simulink model "fan_controller"  (R2020a)
settings: Solver=FixedStepDiscrete  StartTime=0.0  StopTime=10.0  FixedStep=1  RelTol=1e-3
model workspace (MAT data in the model file):
  initial_h = Simulink.Parameter
  initial_h.Value = 50
  initial_h.Description = 'Initial humidity value to preload downsamplers and differentiators/integrators'
  initial_h.DataType = 'auto'
  initial_h.DocUnits = '%'
  initial_h.Dimensions = [1 1]
  initial_t = Simulink.Parameter
  initial_t.Value = 25
  initial_t.Description = 'Initial temperature value to preload downsamplers and differentiators/integrators'
  initial_t.DataType = 'auto'
  initial_t.DocUnits = '°C'
  initial_t.Dimensions = [1 1]
libraries: dspstat3 x4, simulink x2
settings Model: DataDictionary=fan_controller_setup.sldd  OrderedModelArguments=off  Creator=Kalev  LastModifiedBy=Kalev
settings OptimizationCC: EnhancedBackFolding=on  PassReuseOutputArgsAs=Individual arguments  ZeroExternalMemoryAtStartup=off  ZeroInternalMemoryAtStartup=off  OptimizeBlockOrder=speed  DifferentSizesBufferReuse=on  OptimizationCustomize=off  EfficientTunableParamExpr=on
settings DebuggingCC: ParameterTunabilityLossMsg=error
settings HardwareCC: ProdBitPerPointer=32  ProdBitPerSizeT=32  ProdBitPerPtrDiffT=32  ProdLargestAtomicInteger=Integer  ProdLargestAtomicFloat=Double  ProdWordSize=32  ProdHWDeviceType=Custom Processor->Custom Processor
settings SFSimCC: MATLABDynamicMemAlloc=off
settings RTWCC: SystemTargetFile=ert.tlc  GenCodeOnly=on  TemplateMakefile=ert_default_tmf  GenerateReport=on  BuildConfiguration=Debug  LaunchReport=on  TargetLang=C++
settings CodeAppCC: ForceParamTrailComments=on  IgnoreCustomStorageClasses=off  OperatorAnnotations=on  SimulinkDataObjDesc=on  SFDataObjDesc=on  InsertBlockDesc=on
settings ERTTargetCC: TargetLangStandard=C++03 (ISO)  GenerateSampleERTMain=on  MultiInstanceERTCode=on  CodeInterfacePackaging=C++ class  RootIOFormat=Structure reference  ERTCustomFileTemplate=example_file_process.tlc

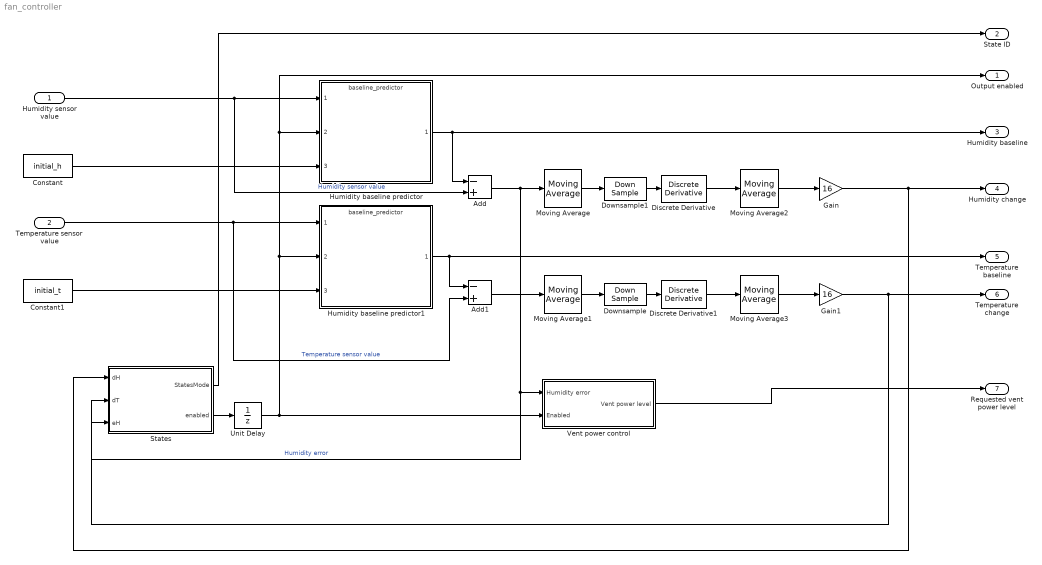
== system fan_controller ==
  Humidity sensor value : Inport
  Temperature sensor value : Inport  Port=2
  Add : Sum  Inputs=-+
  Add1 : Sum  Inputs=-+
  Constant : Constant  Value=initial_h
  Constant1 : Constant  Value=initial_t
  Discrete Derivative : simulink/Discrete/Discrete Derivative  gainval=1.0  ICPrevScaledInput=initial_h  OutMin=[]  OutMax=[]  OutDataType=fixdt(1, 16)  OutScaling=2^-10  DoSatur=off
  Discrete Derivative1 : simulink/Discrete/Discrete Derivative  gainval=1.0  ICPrevScaledInput=initial_t  OutMin=[]  OutMax=[]  OutDataType=fixdt(1, 16)  OutScaling=2^-10  DoSatur=off
  Downsample : DownSample  N=16  phase=15  ic=initial_t
  Downsample1 : DownSample  N=16  phase=15  ic=initial_h
  Gain : Gain  Gain=16
  Gain1 : Gain  Gain=16
  Humidity baseline predictor : ModelReference  ModelNameDialog=baseline_predictor.slx  SimulationMode=Normal  ModelReferenceVersion=1.4
  Humidity baseline predictor1 : ModelReference  ModelNameDialog=baseline_predictor.slx  SimulationMode=Normal  ModelReferenceVersion=1.4
  Moving Average{,1..3} (4 alike) : dspstat3/Moving Average  Method=Sliding window  ForgettingFactorPort=off  SpecifyWindowLength=on  WindowLength=16  ForgettingFactor=0.9  SimulateUsing=Code generation
  States : Stateflow chart  TreatAsAtomicUnit=on
  Unit Delay : UnitDelay  SampleTime=-1  HasFrameUpgradeWarning=on
  Vent power control : Subsystem
  Output enabled : Outport
  State ID : Outport  Port=2
  Humidity baseline : Outport  Port=3
  Humidity change : Outport  Port=4
  Temperature baseline : Outport  Port=5
  Temperature change : Outport  Port=6
  Requested vent power level : Outport  Port=7
  wires:
  Downsample/1 -> Discrete Derivative1/1
  Unit Delay/1 -> Humidity baseline predictor1/2, Output enabled/1, Humidity baseline predictor/2, Vent power control/2(Enabled)
  States/2(enabled) -> Unit Delay/1
  Moving Average1/1 -> Downsample/1
  Vent power control/1(Vent power level) -> Requested vent power level/1
  States/1(StatesMode) -> State ID/1
  Humidity sensor value/1 -> Add/2, Humidity baseline predictor/1  "Humidity sensor value"
  Temperature sensor value/1 -> Add1/2, Humidity baseline predictor1/1  "Temperature sensor value"
  Add1/1 -> Moving Average1/1
  Add/1 -> Moving Average/1, States/3(eH), Vent power control/1(Humidity error)  "Humidity error"
  Discrete Derivative1/1 -> Moving Average3/1
  Moving Average3/1 -> Gain1/1
  Downsample1/1 -> Discrete Derivative/1
  Discrete Derivative/1 -> Moving Average2/1
  Moving Average/1 -> Downsample1/1
  Gain/1 -> Humidity change/1, States/1(dH)
  Humidity baseline predictor1/1 -> Temperature baseline/1, Add1/1
  Moving Average2/1 -> Gain/1
  Gain1/1 -> Temperature change/1, States/2(dT)
  Humidity baseline predictor/1 -> Add/1, Humidity baseline/1
  Constant/1 -> Humidity baseline predictor/3
  Constant1/1 -> Humidity baseline predictor1/3

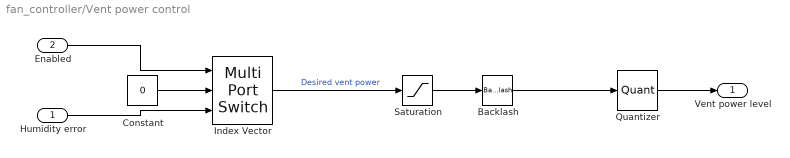
== system fan_controller/Vent power control ==
  Humidity error : Inport
  Enabled : Inport  Port=2
  Backlash : Backlash  BacklashWidth=2
  Constant : Constant  Value=0
  Index Vector : MultiPortSwitch  DataPortOrder=Zero-based contiguous  Inputs=2  zeroidx=on
  Quantizer : Quantizer  QuantizationInterval=30/4  LinearizeAsGain=off
  Saturation : Saturate  UpperLimit=30  LowerLimit=0
  Vent power level : Outport
  wires:
  Constant/1 -> Index Vector/2
  Index Vector/1 -> Saturation/1  "Desired vent power"
  Humidity error/1 -> Index Vector/3
  Enabled/1 -> Index Vector/1
  Quantizer/1 -> Vent power level/1
  Saturation/1 -> Backlash/1
  Backlash/1 -> Quantizer/1

== stateflow chart fan_controller/States ==
  state Stopping
    entry: enabled=0
  state Detected
    entry: enabled=1
  state Stable
    entry: enabled=1
  state OFF
    entry: enabled=0
  Stopping -> OFF
  Detected -> OFF [order 1] : [dH <  -5]
  Stable -> Stopping : [eH < 8]
  (default) -> OFF
  Detected -> Stable [order 2] : [eH > 10]
  OFF -> Detected : [dH > 4]
  data: dH input; dT input; StatesMode output Enum: StatesModeType; enabled output; eH input
